simulink model "testNavigationSolMetrics"  (R2021a)
settings: Solver=VariableStepAuto  StartTime=0.0  StopTime=3600  RelTol=1e-3
libraries: sharedtransform x3
settings Model: Creator=Laura  LastModifiedBy=Laura

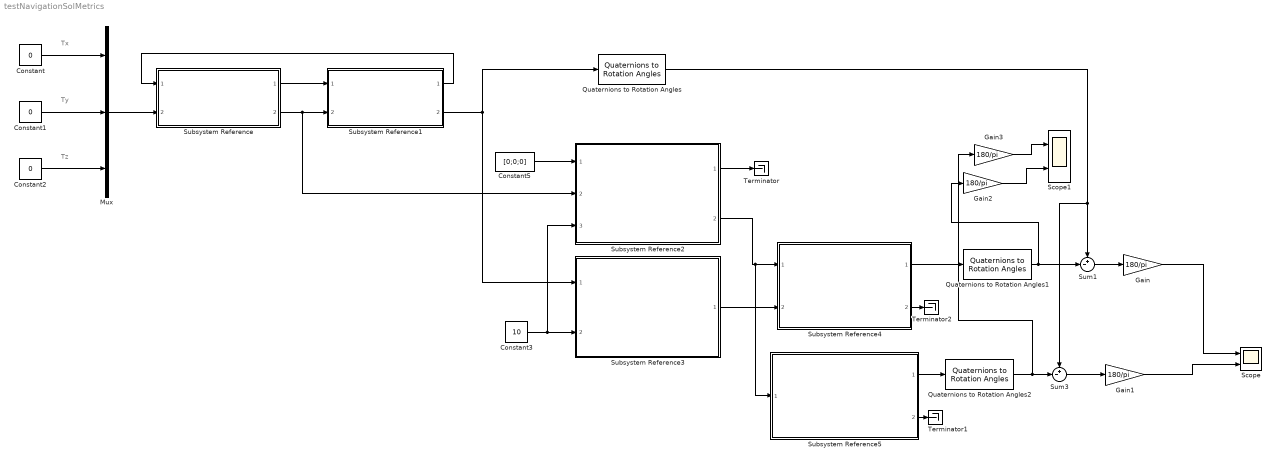
== system testNavigationSolMetrics ==
  note: Tz
  note: Ty
  note: Tx
  Constant : Constant  Value=0
  Constant1 : Constant  Value=0
  Constant2 : Constant  Value=0
  Constant3 : Constant  Value=10
  Constant5 : Constant  Value=[0;0;0]
  Gain{,1..3} (4 alike) : Gain  Gain=180/pi
  Mux : Mux  Inputs=3
  Quaternions to Rotation Angles : sharedtransform/Quaternions to Rotation Angles  rotationOrder=ZYX  aMode=aMode
      settings: SourceProductBaseCode=AE,PW,DR,MT,UV,VE
  Quaternions to Rotation Angles1 : sharedtransform/Quaternions to Rotation Angles  rotationOrder=ZYX  aMode=aMode
      settings: SourceProductBaseCode=AE,PW,DR,MT,UV,VE
  Quaternions to Rotation Angles2 : sharedtransform/Quaternions to Rotation Angles  rotationOrder=ZYX  aMode=aMode
      settings: SourceProductBaseCode=AE,PW,DR,MT,UV,VE
  Scope : Scope  NumInputPorts=2
  Scope1 : Scope  NumInputPorts=2
  Subsystem Reference : Subsystem  ReferencedSubsystem=Dynamics
  Subsystem Reference1 : Subsystem  ReferencedSubsystem=Kinematics
  Subsystem Reference2 : Subsystem  ReferencedSubsystem=IMU
  Subsystem Reference3 : Subsystem  ReferencedSubsystem=StarTracker
  Subsystem Reference4 : Subsystem  ReferencedSubsystem=NavigationSolution
  Subsystem Reference5 : Subsystem  ReferencedSubsystem=InertialNavigationSolution
  Sum1 : Sum  Inputs=+-|
  Sum3 : Sum  Inputs=+-|
  Terminator : Terminator
  Terminator1 : Terminator
  Terminator2 : Terminator
  wires:
  Constant/1 -> Mux/1
  Constant1/1 -> Mux/2
  Subsystem Reference1/1 -> Subsystem Reference/1
  Subsystem Reference/1 -> Subsystem Reference1/1
  Mux/1 -> Subsystem Reference/2
  Constant2/1 -> Mux/3
  Constant3/1 -> Subsystem Reference2/3, Subsystem Reference3/2
  Constant5/1 -> Subsystem Reference2/1
  Subsystem Reference2/1 -> Terminator/1
  Subsystem Reference1/2 -> Quaternions to Rotation Angles/1, Subsystem Reference3/1
  Subsystem Reference/2 -> Subsystem Reference2/2, Subsystem Reference1/2
  Subsystem Reference3/1 -> Subsystem Reference4/2
  Sum1/1 -> Gain/1
  Gain/1 -> Scope/1
  Quaternions to Rotation Angles1/1 -> Gain2/1, Sum1/2
  Subsystem Reference4/1 -> Quaternions to Rotation Angles1/1
  Subsystem Reference2/2 -> Subsystem Reference5/1, Subsystem Reference4/1
  Quaternions to Rotation Angles/1 -> Sum3/1, Sum1/1
  Sum3/1 -> Gain1/1
  Quaternions to Rotation Angles2/1 -> Gain3/1, Sum3/2
  Subsystem Reference5/1 -> Quaternions to Rotation Angles2/1
  Subsystem Reference5/2 -> Terminator1/1
  Subsystem Reference4/2 -> Terminator2/1
  Gain1/1 -> Scope/2
  Gain3/1 -> Scope1/1
  Gain2/1 -> Scope1/2
